simulink model "amk_real_model"  (R2022b)
settings: Solver=FixedStepAuto  StartTime=0.0  StopTime=0.5  FixedStep=1e-6  RelTol=1e-3
values from neighbouring files (symbols this model uses):
  a_fw = log(9)/trfw    [amk_sim.m]    (also in amk_sim_2.m)
  ac = log(9)/tr    [amk_sim.m]    (also in amk_sim_2.m)
  as = log(9)/trs    [amk_sim.m]    (also in amk_sim_2.m)
  ba = 2*k^2*(as*J - 0)/(np^2*psi)    [amk_sim.m]    (also in amk_sim_2.m = 2*k^2*(as*J - bm)/(np^2*psi))
  bm = 0.02    [amk_sim.m]    (also in amk_sim_2.m = 0.008)
  fsw = 8e3    (= 8000)    [amk_sim.m]    (also in amk_sim_2.m)
  I_base = 85.7    [amk_sim.m]    (also in amk_sim_2.m)
  I_max = 85.7    [amk_sim.m]    (also in amk_sim_2.m)
  Icon = 33.5    [amk_sim.m]    (also in amk_sim_2.m)
  Imax_interval = 1.24    [amk_sim.m]    (also in amk_sim_2.m = 5)
  Ipeak = 85.7    [amk_sim.m]    (also in amk_sim_2.m = 87.5)
  J = 2.5*(2.74e-4)    (= 0.000685)    [amk_sim.m]    (also in amk_sim_2.m = 0.000528)
  k = 1    [amk_sim.m]    (also in amk_sim_2.m)
  ki_s = 2*k^2*as^2*J/(np^2*psi)    [amk_sim.m]    (also in amk_sim_2.m)
  kp_s = 2*k^2*as*J/(np^2*psi)    [amk_sim.m]    (also in amk_sim_2.m)
  Ld = Ldm    (= 0.0004)    [amk_sim.m]    (also in amk_sim_2.m = 0.00012)
  Lq = Lqm    (= 0.00052)    [amk_sim.m]    (also in amk_sim_2.m = 0.00024)
  max_temp = 140    [amk_sim.m]    (also in amk_sim_2.m)
  np = 5    [amk_sim.m]    (also in amk_sim_2.m)
  Peak_power = 45000    [amk_sim.m]    (also in amk_sim_2.m = 50000)
  Peak_regen = -15000    [amk_sim.m]    (also in amk_sim_2.m = -1500000)
  psi = 0.047    [amk_sim.m]    (also in amk_sim_2.m = 0.05077789)
  rpm_nom = 20000    [amk_sim.m]    (also in amk_sim_2.m = 12000)
  Rs = 202.5e-3    (= 0.2025)    [amk_sim.m]    (also in amk_sim_2.m)
  sample_time = 1e-4    (= 0.0001)    [amk_sim.m]    (also in amk_sim_2.m = 1e-06)
  temp_threshold = 100    [amk_sim.m]    (also in amk_sim_2.m)
  u_dc = 550    [amk_sim.m]    (also in amk_sim_2.m)
  u_nom = u_dc*k    (= 550)    [amk_sim.m]    (also in amk_sim_2.m)
undefined symbols (not defined in the file or in its folder): Icutoff, rc1, rc2, rc3, rc4, rc5
libraries: spsIGBTDiodeLib x6, simulink x5, spsCurrentMeasurementLib x3, spsSeriesRLCBranchLib x3, spsDCVoltageSourceLib x1, spsPermanentMagnetSynchronousMachineLib x1, dspstat3 x1, spsThreePhaseVIMeasurementLib x1, spsMultimeterLib x1, spsTriangleGeneratorLib x1, sps_lib x1
(part 2 of 4)

== system amk_real_model/Speed Limiter/speed controller1/Subsystem2 ==
  psi : Inport
  Constant : Constant  Value=2*k^2*(as*J)/np^2
  Constant1 : Constant  Value=2*k^2*(as*J)/np^2
  Constant2 : Constant  Value=2*k^2*(as^2*J)/np^2
  Divide : Product  Inputs=*/
  Divide1 : Product  Inputs=*/
  Divide2 : Product  Inputs=*/
  ba : Outport
  kps : Outport  Port=2
  kis : Outport  Port=3
  wires:
  Divide2/1 -> kis/1
  Divide1/1 -> kps/1
  Divide/1 -> ba/1
  [psi] -> Divide2/2
  Constant2/1 -> Divide2/1
  Constant1/1 -> Divide1/1
  [psi] -> Divide1/2
  [psi] -> Divide/2
  psi/1 -> [psi]
  Constant/1 -> Divide/1

== matlab function amk_real_model/pm flux est ==
  data: Iq input; psi output
function psi= fcn(Iq)

pm_flux = [47.22932693 47.21431813 47.05146664	46.75587183	46.34316 45.82916949 45.22964911 44.56000026 43.83468728 43.06630479 42.26389314 41.43526414 40.58848093 39.73068354 38.86734457 38.00279887 37.14115431 36.28662807 35.44396164 34.61891364 33.81865599];

Iq_array = [0	4.28660705	8.573214102	12.85982115	17.1464282	21.43303539	25.71964261	30.00624953	34.29285645	38.57946347	42.86607073	47.15267796	51.4392846	55.72589165	60.01249877	64.29910575	68.58571287	72.87231986	77.1589269	81.44553396	85.732141];

if(Iq > Iq_array(20))
    psi = pm_flux(21)/1000;
else
    i = cast(Iq/4.2866, "uint8");

    low = Iq_array(i+1);

    precentage = (Iq - low)/Iq_array(2);
    
    psi = (precentage*pm_flux(i+2)+(1-precentage)*pm_flux(i+1))/1000;
end

== matlab function amk_real_model/I2t/MATLAB Function ==
  data: u input; y output; t input; c input
function y = fcn(u, t, c)
double k;

if (u > c)
    k = 1;
else
    k = -1;
end

if(t < 0.0001)
    k = 1;
end
y = k;
